simulink model "adv_lag_simulink"  (R2016a)
settings: Solver=VariableStepAuto  StartTime=0.0  StopTime=30  RelTol=1e-3
values from neighbouring files (symbols this model uses):
  Kc = Kp_desejado/Kp_antigo    (= 99)    [adv_lag_igual.m]    (also in advance_and_lagging_compensator.m = (1)/abs(((s1+zero_adv)/(s1+polo_adv))*planta); advance_compensator.m = (1)/abs(((s1+zero_cont1)/(s1+polo_cont1))*planta); lagging_compensator.m = (1)/abs(((s1+zero_lag)/(s1+polo_lag))*planta))
  polo_adv = 39.8730    (= 39.873)    [adv_lag_igual.m]    (also in advance_and_lagging_compensator.m = sigma + wd*tand(-deficiencia_angular))
  polo_lag = 1/(beta*T2)    (= 0.0702229578913)    [adv_lag_igual.m]    (also in advance_and_lagging_compensator.m = 1/(beta*T2); lagging_compensator.m = 1/(beta*T))
  zero_adv = 4    [adv_lag_igual.m]    (also in advance_and_lagging_compensator.m = abs(max(polos_planta)))
  zero_lag = 0.7    [adv_lag_igual.m]    (also in advance_and_lagging_compensator.m = input('Escolha um Zero para o controlador perto da Origem-> ; lagging_compensator.m = input('Escolha um Zero para o controlador PERTO DE ZERO-> '))
settings Model: Creator=jessa  LastModifiedBy=jessa

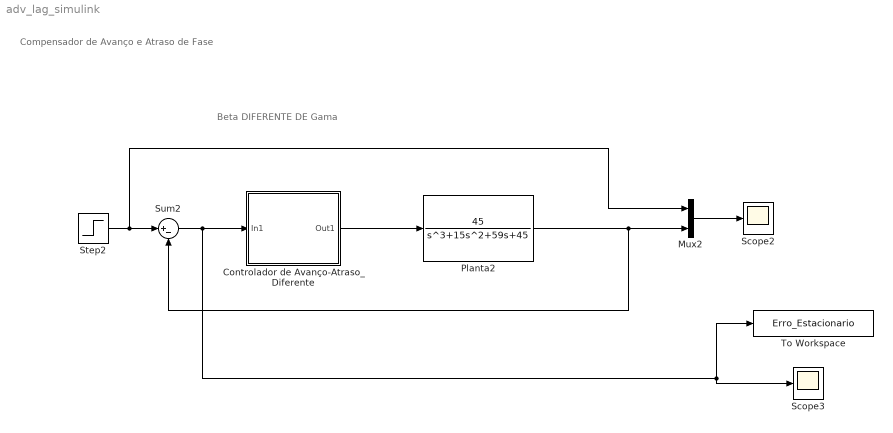
== system adv_lag_simulink ==
  note: Compensador de Avanço e Atraso de Fase
  note: Beta DIFERENTE DE Gama
  Controlador de Avanço-Atraso_Diferente : Subsystem
  Mux2 : Mux  Inputs=2
  Planta2 : TransferFcn  Numerator=[45]  Denominator=[1 15 59 45]
  Scope2 : Scope
  Scope3 : Scope
  Step2 : Step  Time=0  SampleTime=0
  Sum2 : Sum  Inputs=|+-
  To Workspace : ToWorkspace  VariableName=Erro_Estacionario  SampleTime=-1
  wires:
  Mux2/1 -> Scope2/1
  Planta2/1 -> Sum2/2, Mux2/2
  Step2/1 -> Sum2/1, Mux2/1
  Sum2/1 -> To Workspace/1, Scope3/1, Controlador de Avanço-Atraso_Diferente/1(In1)
  Controlador de Avanço-Atraso_Diferente/1(Out1) -> Planta2/1

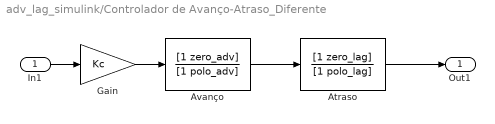
== system adv_lag_simulink/Controlador de Avanço-Atraso_Diferente ==
  In1 : Inport
  Atraso : TransferFcn  Numerator=[1 zero_lag]  Denominator=[1 polo_lag]
  Avanço : TransferFcn  Numerator=[1 zero_adv]  Denominator=[1 polo_adv]
  Gain : Gain  Gain=Kc
  Out1 : Outport
  wires:
  In1/1 -> Gain/1
  Gain/1 -> Avanço/1
  Avanço/1 -> Atraso/1
  Atraso/1 -> Out1/1
